simulink model "demo_env"  (R2024a)
settings: Solver=FixedStepAuto  StartTime=0.0  StopTime=10.0  FixedStep=0.1  RelTol=1e-3
PostLoadFcn:
  | on_model_load
StartFcn:
  | on_model_start
StopFcn:
  | on_simulation_done
undefined symbols (not defined in the file or in its folder): ActiveScenario
libraries: test_lib_ctl x1, test_lib_sys x1
PostSaveFcn:
  | on_model_save
settings Model: Creator=luka  LastModifiedBy=luka

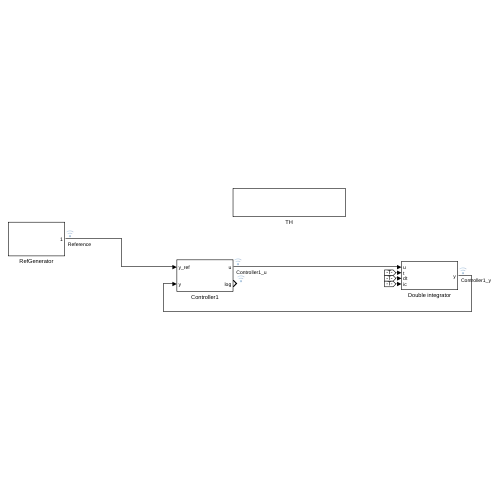
[thumbnail: Simulink's stored preview of the top-level diagram]
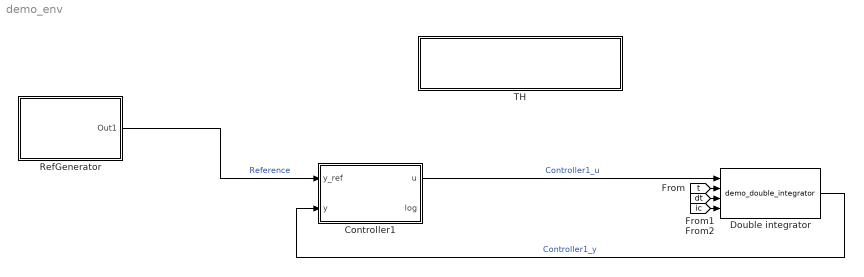
== system demo_env ==
  Controller1 : Subsystem
  Double integrator : test_lib_sys/demo_double_integrator  Tag=__cs_slx_sys;  k1=0  k2=0  iid__=[0]  pid__=[100 101 109 111 95 100 111 117 98 108 101 95 105 110 116 101 103 114 97 116 111 114 58 116 101 115 116 95 108 105 98]  params_struct_name=demo_env_params.sys.DoubleIntegrator
  RefGenerator : Subsystem  mask{scenario=P1}
      settings: OpenFcn=on_reference_generator_open();
      mask TypeOptions scenario: P1
      mask Callback scenario: on_reference_select;
      mask DialogControl edit_refs_btn Prompt: Edit reference
      mask DialogControl edit_refs_btn Callback: on_edit_references_btn;
  TH : Subsystem
      mask DialogControl ParameterGroupVar Prompt: Params
  wires:
  [t] -> Double integrator/2
  [dt] -> Double integrator/3
  [ic] -> Double integrator/4
  Controller1/1(u) -> Double integrator/1  "Controller1_u"
  Double integrator/1 -> Controller1/2(y)  "Controller1_y"
  RefGenerator/1(Out1) -> Controller1/1(y_ref)  "Reference"

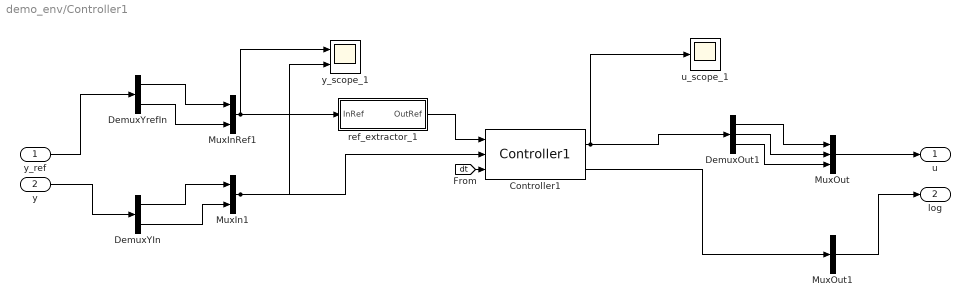
== system demo_env/Controller1 ==
  y_ref : Inport  PortDimensions=2
  y : Inport  Port=2  PortDimensions=2
  Controller1 : test_lib_ctl/Controller1  Tag=__cs_m_ctl;  iid__=[0]  pid__=[67 111 110 116 114 111 108 108 101 114 49 58 116 101 115 116 95 108 105 98]  LogEntryType=Controller1_LT  params=demo_env_params.ctl.Controller1  data=Controller1_data  ParamsType=Controller1_PT  DataType=Controller1_DT  u_ic=0
  DemuxOut1 : Demux  Outputs=3
  DemuxYIn : Demux  Outputs=2
  DemuxYrefIn : Demux  Outputs=2
  MuxIn1 : Mux  Inputs=2
  MuxInRef1 : Mux  Inputs=2
  MuxOut : Mux  Inputs=3
  MuxOut1 : BusCreator  Inputs=1
  ref_extractor_1 : Subsystem
  u_scope_1 : Scope
  y_scope_1 : Scope  NumInputPorts=2
  u : Outport  PortDimensions=3
  log : Outport  Port=2
  wires:
  [dt] -> Controller1/3
  y/1 -> DemuxYIn/1
  y_ref/1 -> DemuxYrefIn/1
  MuxOut/1 -> u/1
  MuxOut1/1 -> log/1
  MuxInRef1/1 -> ref_extractor_1/1(InRef), y_scope_1/1
  ref_extractor_1/1(OutRef) -> Controller1/1
  MuxIn1/1 -> Controller1/2, y_scope_1/2
  Controller1/1 -> DemuxOut1/1, u_scope_1/1
  Controller1/2 -> MuxOut1/1
  DemuxYIn/1 -> MuxIn1/1
  DemuxYrefIn/1 -> MuxInRef1/1
  DemuxYIn/2 -> MuxIn1/2
  DemuxYrefIn/2 -> MuxInRef1/2
  DemuxOut1/1 -> MuxOut/1
  DemuxOut1/2 -> MuxOut/2
  DemuxOut1/3 -> MuxOut/3

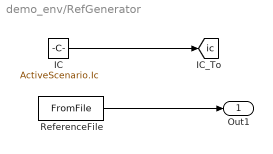
== system demo_env/RefGenerator ==
  IC : Constant  Value=ActiveScenario.Ic
  ReferenceFile : FromFile  SampleTime=0
  Out1 : Outport
  tag scope: ic=global
  wires:
  IC/1 -> [ic]
  ReferenceFile/1 -> Out1/1

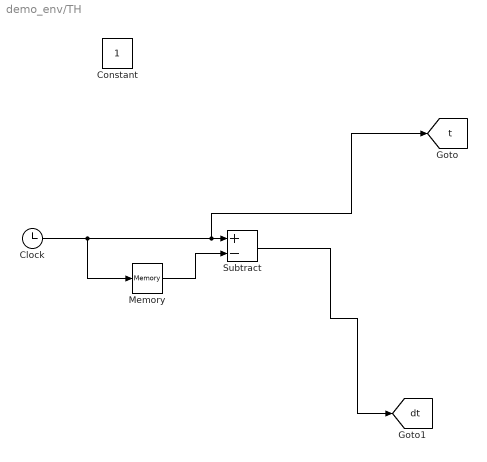
== system demo_env/TH ==
  Clock : Clock
  Constant : Constant
  Memory : Memory
  Subtract : Sum  Inputs=+-
  tag scope: dt=global, t=global
  wires:
  Subtract/1 -> [dt]
  Memory/1 -> Subtract/2
  Clock/1 -> Memory/1, Subtract/1, [t]

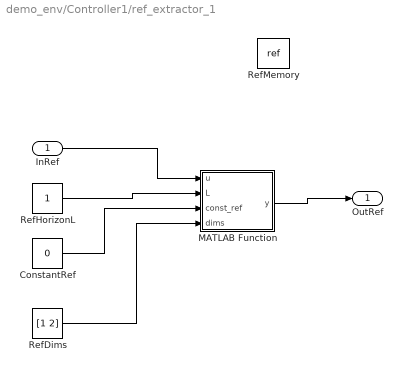
== system demo_env/Controller1/ref_extractor_1 ==
  InRef : Inport
  ConstantRef : Constant  Value=0
  MATLAB Function : MATLAB Function  TreatAsAtomicUnit=on
  RefDims : Constant  Value=[1 2]
  RefHorizonL : Constant
  RefMemory : DataStoreMemory  DataStoreName=ref  WriteAfterWriteMsg=warning  ShowAdditionalParam=off  OutDataTypeStr=double
  OutRef : Outport
  wires:
  ConstantRef/1 -> MATLAB Function/3(const_ref)
  RefDims/1 -> MATLAB Function/4(dims)
  RefHorizonL/1 -> MATLAB Function/2(L)
  InRef/1 -> MATLAB Function/1(u)
  MATLAB Function/1(y) -> OutRef/1

== matlab function demo_env/Controller1/ref_extractor_1/MATLAB Function ==
  settings: updateMethod=DISCRETE
  data: u input; L input; const_ref input; dims input; y output; ref data_store_memory; GlobalReference parameter
function y = fcn(u, L, const_ref, dims, GlobalReference)

persistent cnt
global ref

if isempty(cnt)
    cnt = 0;
end
cnt = cnt+1;

horizon_end = cnt+L-1;
if L > 1 
   if horizon_end > length(GlobalReference)
        if size(ref, 1) == size(u, 1)
            y = permute(ref, [2, 1]);
        else
            y = ref;
        end       
        return
   end

   if size(ref, 1) == size(u, 1)
      
      if const_ref == 0
        ref(:, :) = GlobalReference(cnt:horizon_end, dims)';
      else
        ref(:, :) = repmat(GlobalReference(cnt, dims)', 1, L);
      end
      y = permute(ref, [2, 1]);
   else
      if const_ref == 0
        ref(1:L, :) = GlobalReference(cnt:horizon_end, dims);
      else
        ref(1:L, :) = repmat(GlobalReference(cnt, dims), L, 1);
      end
      y = ref;
   end
else
   if size(ref, 1) == size(u, 1)
       ref = u;
       y = permute(ref, [2, 1]);
   else
      ref(1, :) = u';
      y = ref;
   end
end
